simulink model "BLDCctrlBasedOnMBD"  (R2020b)
settings: Solver=FixedStepDiscrete  StartTime=0.0  StopTime=10.0  FixedStep=0.0001  RelTol=1e-3
PreLoadFcn:
  | load('structBLDCMotorCrtl.mat');
InitFcn:
  | mbd_s32k_consistency_checks(bdroot(gcs));
undefined symbols (not defined in the file): External, LQFP, One, Shot, TRGMUX_PDB_TRIG
libraries: mbd_s32k1xx_ec_toolbox x34, mcbcontrolslib x4, mbd_msd_ec_toolbox x1
(part 2 of 2)

== matlab function BLDCctrlBasedOnMBD/State Machine Task/State Functions/NomalRunFunc/Truth Table ==
  data: Hallsum input uint8; DutyA output single; DutyB output single; DutyC output single; DutyReq input single; SWOCTRLcode output uint16; OUTMASKcode output uint8
function [DutyA, DutyB, DutyC, SWOCTRLcode, OUTMASKcode] = fcn(Hallsum, DutyReq)

aVarTruthTableCondition_1 = false;
aVarTruthTableCondition_2 = false;
aVarTruthTableCondition_3 = false;
aVarTruthTableCondition_4 = false;
aVarTruthTableCondition_5 = false;
aVarTruthTableCondition_6 = false;


% Condition #1
aVarTruthTableCondition_1 = logical(Hallsum == 1);

% Condition #2
aVarTruthTableCondition_2 = logical(Hallsum == 2);

% Condition #3
aVarTruthTableCondition_3 = logical(Hallsum == 3);

% Condition #4
aVarTruthTableCondition_4 = logical(Hallsum == 4);

% Condition #5
aVarTruthTableCondition_5 = logical(Hallsum == 5);

% Condition #6
aVarTruthTableCondition_6 = logical(Hallsum == 6);

if (aVarTruthTableCondition_1 && ~aVarTruthTableCondition_2 && ~aVarTruthTableCondition_3 && ~aVarTruthTableCondition_4 && ~aVarTruthTableCondition_5 && ~aVarTruthTableCondition_6)
    aFcnTruthTableAction_1();
elseif (~aVarTruthTableCondition_1 && aVarTruthTableCondition_2 && ~aVarTruthTableCondition_3 && ~aVarTruthTableCondition_4 && ~aVarTruthTableCondition_5 && ~aVarTruthTableCondition_6)
    aFcnTruthTableAction_2();
elseif (~aVarTruthTableCondition_1 && ~aVarTruthTableCondition_2 && aVarTruthTableCondition_3 && ~aVarTruthTableCondition_4 && ~aVarTruthTableCondition_5 && ~aVarTruthTableCondition_6)
    aFcnTruthTableAction_3();
elseif (~aVarTruthTableCondition_1 && ~aVarTruthTableCondition_2 && ~aVarTruthTableCondition_3 && aVarTruthTableCondition_4 && ~aVarTruthTableCondition_5 && ~aVarTruthTableCondition_6)
    aFcnTruthTableAction_4();
elseif (~aVarTruthTableCondition_1 && ~aVarTruthTableCondition_2 && ~aVarTruthTableCondition_3 && ~aVarTruthTableCondition_4 && aVarTruthTableCondition_5 && ~aVarTruthTableCondition_6)
    aFcnTruthTableAction_5();
elseif (~aVarTruthTableCondition_1 && ~aVarTruthTableCondition_2 && ~aVarTruthTableCondition_3 && ~aVarTruthTableCondition_4 && ~aVarTruthTableCondition_5 && aVarTruthTableCondition_6)
    aFcnTruthTableAction_6();
else % Default
    aFcnTruthTableAction_7();
end

function aFcnTruthTableAction_1()

% Example action 1 called from D1 & D2 column in condition table

DutyA = DutyReq;
DutyB = 0;
DutyC = 0;
SWOCTRLcode = 0x2020;
OUTMASKcode = 0x1C;

function aFcnTruthTableAction_2()

% Example action 2 called from D3 column in condition table

DutyA = 0;
DutyB = DutyReq;
DutyC = 0;
SWOCTRLcode = 0x0202;
OUTMASKcode = 0x31;

function aFcnTruthTableAction_3()



DutyA = 0;
DutyB = DutyReq;
DutyC = 0;
SWOCTRLcode = 0x2020;
OUTMASKcode =0x13;

function aFcnTruthTableAction_4()



DutyA = 0;
DutyB = 0;
DutyC = DutyReq;
SWOCTRLcode = 0x0808;
OUTMASKcode =0x07;

function aFcnTruthTableAction_5()



DutyA = DutyReq;
DutyB = 0;
DutyC = 0;
SWOCTRLcode = 0x0808;
OUTMASKcode =0x34;

function aFcnTruthTableAction_6()



DutyA = 0;
DutyB = 0;
DutyC = DutyReq;
SWOCTRLcode = 0x0202;
OUTMASKcode =0x0D;

function aFcnTruthTableAction_7()



DutyA = 0;
DutyB = 0;
DutyC = 0;
SWOCTRLcode = 0x0000;
OUTMASKcode =0x3F;

== stateflow chart BLDCctrlBasedOnMBD/State Machine Task/Chart ==
  state ReadADC [parallel]
    ReadADCFunc;
    settings: executionOrder=1
  state StateMachine [parallel]
    settings: executionOrder=2
    state Initial
      en:
      InitFunc;
      InitDone = true;
      bind:InitFunc;
    state Ready
      en:ReadyFunc;
      du:ReadyFunc;
      bind:ReadyFunc;
    state Run
      MeasFunc;
      state Calibration
        en:CalCnt = 0;
        du:CalCnt = CalCnt + 1;CalFunc;
        bind:CalFunc;
      state NormalRun
        en:NormalRunFunc;
        du:NormalRunFunc;
        bind:NormalRunFunc;
      (default) -> Calibration
      Calibration -> NormalRun : [CalCnt > 10000]{CalCnt = 0;}
    state Faults
      en:FaultFunc;
      du:FaultFunc;
      bind:FaultFunc;
    Run -> Initial [order 1] : [~MotorOnOff]{InitDone = false;}
    (default) -> Initial : {InitDone = false;}
    Initial -> Ready [order 1] : [InitDone]
    Ready -> Run [order 1] : [MotorOnOff]
    Ready -> Faults [order 2] : [FaultSetClear]
    Faults -> Initial : [~FaultSetClear]
    Initial -> Faults [order 2] : [FaultSetClear]
    Run -> Faults [order 2] : [FaultSetClear]
  state UpdateFTM [parallel]
    UpdateFTMFunc;
    settings: executionOrder=3
  data: CalCnt local; InitDone local boolean; MotorOnOff input boolean; FaultSetClear input boolean
  events: MeasFunc output FUNCTION_CALL_EVENT; InitFunc output FUNCTION_CALL_EVENT; ReadyFunc output FUNCTION_CALL_EVENT; CalFunc output FUNCTION_CALL_EVENT; NormalRunFunc output FUNCTION_CALL_EVENT; FaultFunc output FUNCTION_CALL_EVENT; ReadADCFunc output FUNCTION_CALL_EVENT; UpdateFTMFunc output FUNCTION_CALL_EVENT
